simulink model "ESP32_UDP_UART_Bridge"  (R2024b)
settings: Solver=ode4  StartTime=0.0  StopTime=Inf  FixedStep=0.005  RelTol=1e-3  EnableMultiTasking=on
values from neighbouring files (symbols this model uses):
  UDP_DIAG_SOURCE_ID = uint8(1)    [ESP32_UDP_UART_Setup.m]
libraries: arduinowifilib x1, arduinolib x1
(part 2 of 3)

== matlab function ESP32_UDP_UART_Bridge/MATLAB Function3 ==
  data: now_ms input; safe_status_u8 output; fused_status_u8 input; fused_time_u32 input; fused_pose_f32 input; safe_time_u32 output; safe_cmd_u8 output; safe_pose_f32 output
% =========================================================
% ESP32_Link_Safety
% =========================================================
% Zadanie:
%   Realizuje warstwę bezpieczeństwa łącza Vision po fuzji pomiarów.
%   Blok decyduje, czy można dalej jechać, czy należy utrzymać ostatni
%   stan, zmniejszać speed, albo wykonać hard stop.
%
% Wejścia:
%   now_ms          : lokalny czas ESP32 w ms, uint32
%   fused_status_u8 : status z Vision_Measurement_Fusion, 8x1
%   fused_time_u32  : czasy z Vision_Measurement_Fusion, 3x1
%   fused_pose_f32  : pozycja fused, 6x1
%
% Wyjścia:
%   safe_status_u8, 8x1:
%     1 = pose_valid
%     2 = deadman_out
%     3 = move_en_out
%     4 = safe_to_drive
%     5 = hold_mode
%     6 = soft_decay
%     7 = hard_stop
%     8 = source_id
%
%   safe_time_u32, 3x1:
%     1 = seq
%     2 = unity_t_ms
%     3 = link_age_ms
%
%   safe_cmd_u8, 2x1:
%     1 = speed_pct
%     2 = fps_hz
%
%   safe_pose_f32, 6x1:
%     1 = x_m
%     2 = y_m
%     3 = z_m
%     4 = yaw_deg
%     5 = yaw_deg_unwrapped
%     6 = yaw_rate_dps
%
% Metodyka:
%   Jeśli fused_available=1, blok zapamiętuje ostatni poprawny stan.
%   Jeśli przez krótki czas nie ma nowego fused state, blok korzysta
%   z ostatniego zapamiętanego stanu i przechodzi przez tryby:
%      0..75 ms    : normal
%      75..150 ms  : hold last
%      150..250 ms : soft decay, liniowe zmniejszanie speed_pct
%      >250 ms     : hard stop
%
%   Jeśli operator_stop_request=1, hard stop wykonywany jest natychmiast,
%   bez czekania na timeout.
%
% Uwagi:
%   Ten blok nie dekoduje UDP i nie wybiera źródła. Jego zadaniem jest
%   wyłącznie bezpieczne zachowanie wyjścia przy utracie lub zatrzymaniu
%   danych Vision.
% =========================================================

function [safe_status_u8, safe_time_u32, safe_cmd_u8, safe_pose_f32] = ESP32_Link_Safety(now_ms, fused_status_u8, fused_time_u32, fused_pose_f32)
%#codegen

HOLD_NORMAL_MS = uint32(75);
HOLD_LAST_MS   = uint32(150);
SOFT_STOP_MS   = uint32(250);

safe_status_u8 = zeros(8, 1, 'uint8');
safe_time_u32  = zeros(3, 1, 'uint32');
safe_cmd_u8    = zeros(2, 1, 'uint8');
safe_pose_f32  = zeros(6, 1, 'single');

persistent has_last last_ms
persistent last_status last_time last_cmd last_pose

if isempty(has_last)
    has_last = uint8(0);
    last_ms = uint32(0);

    last_status = zeros(8, 1, 'uint8');
    last_time   = zeros(3, 1, 'uint32');
    last_cmd    = zeros(2, 1, 'uint8');
    last_pose   = zeros(6, 1, 'single');
end

fused_available = fused_status_u8(1);
operator_stop_request = fused_status_u8(2);

% Świeży stop operatora: deadman/move_en puszczony
if operator_stop_request ~= 0
    safe_status_u8(7) = uint8(1); % hard_stop
    return;
end

% Aktualizacja ostatniego poprawnego fused state
if fused_available ~= 0
    has_last = uint8(1);
    last_ms = now_ms;

    last_status(:) = fused_status_u8(:);
    last_time(:) = fused_time_u32(:);

    last_cmd(1) = fused_status_u8(4); % speed_pct
    last_cmd(2) = fused_status_u8(5); % fps_hz

    last_pose(:) = fused_pose_f32(:);
end

if has_last == 0
    safe_status_u8(7) = uint8(1); % hard_stop
    return;
end

if now_ms >= last_ms
    link_age_ms = now_ms - last_ms;
else
    link_age_ms = uint32(0);
end

safe_status_u8(1) = uint8(1); % pose_valid
safe_status_u8(2) = uint8(1); % deadman_out
safe_status_u8(3) = uint8(1); % move_en_out
safe_status_u8(8) = last_status(3); % source_id

safe_time_u32(1) = last_time(1); % seq
safe_time_u32(2) = last_time(2); % unity_t_ms
safe_time_u32(3) = link_age_ms;

safe_cmd_u8(1) = last_cmd(1); % speed
safe_cmd_u8(2) = last_cmd(2); % fps

safe_pose_f32(:) = last_pose(:);

if link_age_ms <= HOLD_NORMAL_MS
    safe_status_u8(4) = uint8(1); % safe_to_drive

elseif link_age_ms <= HOLD_LAST_MS
    safe_status_u8(4) = uint8(1);
    safe_status_u8(5) = uint8(1); % hold_mode

elseif link_age_ms <= SOFT_STOP_MS
    safe_status_u8(4) = uint8(1);
    safe_status_u8(6) = uint8(1); % soft_decay

    decay_range = double(SOFT_STOP_MS - HOLD_LAST_MS);
    decay_age = double(link_age_ms - HOLD_LAST_MS);
    factor = 1.0 - decay_age / decay_range;

    if factor < 0.0
        factor = 0.0;
    end

    safe_cmd_u8(1) = uint8(double(last_cmd(1)) * factor);

else
    safe_status_u8(:) = uint8(0);
    safe_status_u8(7) = uint8(1); % hard_stop

    safe_time_u32(1) = last_time(1);
    safe_time_u32(2) = last_time(2);
    safe_time_u32(3) = link_age_ms;

    safe_cmd_u8(:) = uint8(0);
    safe_pose_f32(:) = last_pose(:);
end

== matlab function ESP32_UDP_UART_Bridge/ATU1_UART_Frame_Builder ==
  data: safe_status_u8 input; uart_bytes output; safe_time_u32 input; safe_cmd_u8 input; safe_pose_f32 input; uart_debug_u8 output; uart_crc_u16 output
function [uart_bytes, uart_debug_u8, uart_crc_u16] = ATU1_UART_Frame_Builder(safe_status_u8, safe_time_u32, safe_cmd_u8, safe_pose_f32)
%#codegen
% =========================================================
% ATU1_UART_Frame_Builder
% =========================================================
% Zadanie:
%   Buduje binarną ramkę UART ATU1 wysyłaną z ESP32 do STM32.
%   Ramka zawiera przefiltrowany/fused stan Vision oraz flagi safety.
%
% Format wyjściowy ATU1:
%   bajty 1-2   : header 0xA5 0x5A
%   bajt 3      : version = 1
%   bajt 4      : source_id
%   bajty 5-8   : seq uint32 little-endian
%   bajty 9-12  : unity_t_ms uint32 little-endian
%   bajt 13     : flags
%                 bit0 = pose_valid
%                 bit1 = deadman
%                 bit2 = move_en
%                 bit3 = selected/fused data ok
%                 bit4 = safe_to_drive
%                 bit5 = hold_mode
%                 bit6 = soft_decay
%                 bit7 = hard_stop
%   bajt 14     : speed_pct
%   bajt 15     : fps_hz
%   bajt 16     : reserved
%   bajty 17-20 : x_m single little-endian
%   bajty 21-24 : y_m single little-endian
%   bajty 25-28 : z_m single little-endian
%   bajty 29-32 : yaw_deg_unwrapped single little-endian
%   bajty 33-36 : yaw_rate_dps single little-endian
%   bajty 37-38 : crc16 uint16 little-endian
%
% Wejścia:
%   safe_status_u8, 8x1:
%     1 = pose_valid
%     2 = deadman
%     3 = move_en
%     4 = safe_to_drive
%     5 = hold_mode
%     6 = soft_decay
%     7 = hard_stop
%     8 = source_id
%
%   safe_time_u32, 3x1:
%     1 = seq
%     2 = unity_t_ms
%     3 = link_age_ms, nie jest wysyłane w ATU1 V1
%
%   safe_cmd_u8, 2x1:
%     1 = speed_pct
%     2 = fps_hz
%
%   safe_pose_f32, 6x1:
%     1 = x_m
%     2 = y_m
%     3 = z_m
%     4 = yaw_deg, nie jest wysyłane w ATU1 V1
%     5 = yaw_deg_unwrapped
%     6 = yaw_rate_dps
%
% Wyjścia:
%   uart_bytes, 38x1 uint8:
%     gotowa ramka do wysłania przez UART do STM32
%
%   uart_debug_u8, 8x1 uint8:
%     1 = header byte 1
%     2 = header byte 2
%     3 = version
%     4 = source_id
%     5 = flags
%     6 = speed_pct
%     7 = fps_hz
%     8 = frame length
%
%   uart_crc_u16, 1x1 uint16:
%     CRC16 policzone dla ramki ATU1 po bajtach 1..36
%
% Metodyka:
%   Blok mapuje status safety na pole flags, wpisuje wartości liczbowe
%   w kolejności little-endian, a następnie liczy CRC16 CCITT-FALSE
%   po bajtach 1..36. CRC jest zapisywane w bajtach 37..38.
% =========================================================

uart_bytes    = zeros(38, 1, 'uint8');
uart_debug_u8 = zeros(8, 1, 'uint8');
uart_crc_u16  = zeros(1, 1, 'uint16');

pose_valid    = safe_status_u8(1);
deadman       = safe_status_u8(2);
move_en       = safe_status_u8(3);
safe_to_drive = safe_status_u8(4);
hold_mode     = safe_status_u8(5);
soft_decay    = safe_status_u8(6);
hard_stop     = safe_status_u8(7);
source_id     = safe_status_u8(8);

seq        = safe_time_u32(1);
unity_t_ms = safe_time_u32(2);

speed_pct = safe_cmd_u8(1);
fps_hz    = safe_cmd_u8(2);

x_m = safe_pose_f32(1);
y_m = safe_pose_f32(2);
z_m = safe_pose_f32(3);

yaw_deg_unwrapped = safe_pose_f32(5);
yaw_rate_dps      = safe_pose_f32(6);

% Header
uart_bytes(1) = uint8(165); % 0xA5
uart_bytes(2) = uint8(90);  % 0x5A
uart_bytes(3) = uint8(1);   % version
uart_bytes(4) = source_id;

% seq uint32 little-endian
uart_bytes(5) = uint8(bitand(seq, uint32(255)));
uart_bytes(6) = uint8(bitand(bitshift(seq, -8), uint32(255)));
uart_bytes(7) = uint8(bitand(bitshift(seq, -16), uint32(255)));
uart_bytes(8) = uint8(bitand(bitshift(seq, -24), uint32(255)));

% unity_t_ms uint32 little-endian
uart_bytes(9)  = uint8(bitand(unity_t_ms, uint32(255)));
uart_bytes(10) = uint8(bitand(bitshift(unity_t_ms, -8), uint32(255)));
uart_bytes(11) = uint8(bitand(bitshift(unity_t_ms, -16), uint32(255)));
uart_bytes(12) = uint8(bitand(bitshift(unity_t_ms, -24), uint32(255)));

% Flags
flags = uint8(0);

if pose_valid ~= 0
    flags = bitor(flags, uint8(1));    % bit0 pose_valid
end

if deadman ~= 0
    flags = bitor(flags, uint8(2));    % bit1 deadman
end

if move_en ~= 0
    flags = bitor(flags, uint8(4));    % bit2 move_en
end

if pose_valid ~= 0
    flags = bitor(flags, uint8(8));    % bit3 selected/fused data ok
end

if safe_to_drive ~= 0
    flags = bitor(flags, uint8(16));   % bit4 safe_to_drive
end

if hold_mode ~= 0
    flags = bitor(flags, uint8(32));   % bit5 hold_mode
end

if soft_decay ~= 0
    flags = bitor(flags, uint8(64));   % bit6 soft_decay
end

if hard_stop ~= 0
    flags = bitor(flags, uint8(128));  % bit7 hard_stop
end

uart_bytes(13) = flags;
uart_bytes(14) = speed_pct;
uart_bytes(15) = fps_hz;
uart_bytes(16) = uint8(0); % reserved

% x_m single little-endian
b = typecast(single(x_m), 'uint8');
uart_bytes(17) = b(1);
uart_bytes(18) = b(2);
uart_bytes(19) = b(3);
uart_bytes(20) = b(4);

% y_m single little-endian
b = typecast(single(y_m), 'uint8');
uart_bytes(21) = b(1);
uart_bytes(22) = b(2);
uart_bytes(23) = b(3);
uart_bytes(24) = b(4);

% z_m single little-endian
b = typecast(single(z_m), 'uint8');
uart_bytes(25) = b(1);
uart_bytes(26) = b(2);
uart_bytes(27) = b(3);
uart_bytes(28) = b(4);

% yaw_deg_unwrapped single little-endian
b = typecast(single(yaw_deg_unwrapped), 'uint8');
uart_bytes(29) = b(1);
uart_bytes(30) = b(2);
uart_bytes(31) = b(3);
uart_bytes(32) = b(4);

% yaw_rate_dps single little-endian
b = typecast(single(yaw_rate_dps), 'uint8');
uart_bytes(33) = b(1);
uart_bytes(34) = b(2);
uart_bytes(35) = b(3);
uart_bytes(36) = b(4);

% CRC16 CCITT-FALSE po bajtach 1..36
crc = crc16_ccitt_false_36bytes(uart_bytes);

uart_bytes(37) = uint8(bitand(crc, uint16(255)));
uart_bytes(38) = uint8(bitand(bitshift(crc, -8), uint16(255)));

uart_crc_u16(1) = crc;

% Debug
uart_debug_u8(1) = uart_bytes(1);   % 0xA5
uart_debug_u8(2) = uart_bytes(2);   % 0x5A
uart_debug_u8(3) = uart_bytes(3);   % version
uart_debug_u8(4) = uart_bytes(4);   % source_id
uart_debug_u8(5) = uart_bytes(13);  % flags
uart_debug_u8(6) = uart_bytes(14);  % speed_pct
uart_debug_u8(7) = uart_bytes(15);  % fps_hz
uart_debug_u8(8) = uint8(38);       % frame length
end

function crc = crc16_ccitt_false_36bytes(data)
%#codegen

crc = uint16(65535); % 0xFFFF

for i = 1:36
    crc = bitxor(crc, bitshift(uint16(data(i)), 8));

    for b = 1:8
        if bitand(crc, uint16(32768)) ~= 0 % 0x8000
            crc = bitxor(bitshift(crc, 1), uint16(4129)); % 0x1021
        else
            crc = bitshift(crc, 1);
        end
    end
end
end

== matlab function ESP32_UDP_UART_Bridge/UDP_Link_Diagnostics ==
  data: now_ms input; diag_selected_u32 output; debug_source_id input; portA_udp_data input; portA_udp_size input; portB_udp_data input; portB_udp_size input; diag_selected_u8 output; diag_summary_u32 output; diag_src_u32 output; diag_src_u8 output; diag_port_u32 output
function [diag_selected_u32, diag_selected_u8, diag_summary_u32, diag_src_u32, diag_src_u8, diag_port_u32] = ...
    UDP_Link_Diagnostics(now_ms, debug_source_id, ...
    portA_udp_data, portA_udp_size, ...
    portB_udp_data, portB_udp_size)
%#codegen
% =========================================================
% UDP_Link_Diagnostics
% =========================================================
% Zadanie:
%   Równoległa diagnostyka jakości linku UDP Unity -> ESP32.
%   Blok NIE wpływa na tor sterowania/safety. Czyta surowe dane UDP
%   z PortA/PortB, sam sprawdza ramkę ATB1 i liczy statystyki per source_id.
%
% Wejścia:
%   now_ms          - lokalny czas ESP32/symulacji [ms], uint32
%   debug_source_id - source_id 1..4 wybrany do łatwego podglądu
%   portA_udp_data  - Data z WiFi UDP Receive PortA
%   portA_udp_size  - Size z WiFi UDP Receive PortA
%   portB_udp_data  - Data z WiFi UDP Receive PortB
%   portB_udp_size  - Size z WiFi UDP Receive PortB
%
% Wyjścia:
%   diag_selected_u32 - 20x1 statystyki wybranego source_id
%   diag_selected_u8  - 8x1 flagi wybranego source_id
%   diag_summary_u32  - 12x1 podsumowanie wszystkich source_id
%   diag_src_u32      - 20x4 pełne statystyki source_id 1..4
%   diag_src_u8       - 8x4 pełne flagi source_id 1..4
%   diag_port_u32     - 8x2 statystyki PortA/PortB
%
% Zasada sesji:
%   Jeśli przerwa od ostatniej poprawnej ramki source_id > 2000 ms,
%   zaczynamy nową sesję i NIE liczymy tej przerwy jako packet loss.
%
% Zasada świeżości:
%   Źródło jest fresh, jeśli age_ms <= 300 ms.
%
% Format ATB1:
%   42 B, header A1 1A, version=1, source_id=1..4,
%   CRC16/CCITT-FALSE po bajtach 1..40.
% =========================================================

FRESH_MS = uint32(300);
SESSION_GAP_MS = uint32(2000);

persistent src_u32 src_u8 port_u32

if isempty(src_u32)
    src_u32  = zeros(20, 4, 'uint32');
    src_u8   = zeros(8, 4, 'uint8');
    port_u32 = zeros(8, 2, 'uint32');
end

[src_u32, src_u8, port_u32] = update_one_port(now_ms, uint8(1), portA_udp_data, portA_udp_size, src_u32, src_u8, port_u32, SESSION_GAP_MS);
[src_u32, src_u8, port_u32] = update_one_port(now_ms, uint8(2), portB_udp_data, portB_udp_size, src_u32, src_u8, port_u32, SESSION_GAP_MS);

% Aktualizacja age/fresh/in_session dla każdego source_id
for i = 1:4
    if src_u8(1, i) ~= uint8(0)
        last_rx_ms = src_u32(9, i);

        if now_ms >= last_rx_ms
            age_ms = now_ms - last_rx_ms;
        else
            age_ms = uint32(0);
        end

        src_u32(19, i) = age_ms; % age_ms

        if age_ms <= FRESH_MS
            src_u8(2, i) = uint8(1); % fresh_300ms
        else
            src_u8(2, i) = uint8(0);
        end

        if age_ms <= SESSION_GAP_MS
            src_u8(3, i) = uint8(1); % in_session
        else
            src_u8(3, i) = uint8(0);
        end
    end
end

% Summary
diag_summary_u32 = zeros(12, 1, 'uint32');

total_rx_ok = uint32(0);
total_lost = uint32(0);
total_crc_bad = uint32(0);
total_dup = uint32(0);
sources_seen_mask = uint32(0);
fresh_sources_mask = uint32(0);
max_gap_all = uint32(0);
worst_age = uint32(0);
fresh_count = uint32(0);
total_sessions = uint32(0);

for i = 1:4
    total_rx_ok = total_rx_ok + src_u32(1, i);
    total_crc_bad = total_crc_bad + src_u32(2, i);
    total_lost = total_lost + src_u32(3, i);
    total_dup = total_dup + src_u32(4, i);
    total_sessions = total_sessions + src_u32(15, i);

    if src_u8(1, i) ~= uint8(0)
        sources_seen_mask = bitor(sources_seen_mask, bitshift(uint32(1), i - 1));
    end

    if src_u8(2, i) ~= uint8(0)
        fresh_sources_mask = bitor(fresh_sources_mask, bitshift(uint32(1), i - 1));
        fresh_count = fresh_count + uint32(1);
    end

    if src_u32(11, i) > max_gap_all
        max_gap_all = src_u32(11, i);
    end

    if src_u32(19, i) > worst_age
        worst_age = src_u32(19, i);
    end
end

diag_summary_u32(1) = total_rx_ok;
diag_summary_u32(2) = total_lost;
diag_summary_u32(3) = total_crc_bad;
diag_summary_u32(4) = total_dup;
diag_summary_u32(5) = sources_seen_mask;
diag_summary_u32(6) = fresh_sources_mask;
diag_summary_u32(7) = max_gap_all;
diag_summary_u32(8) = worst_age;

den = total_rx_ok + total_lost;
if den > uint32(0)
    diag_summary_u32(9) = uint32((double(total_lost) * 1000.0) / double(den)); % total_loss_permille
else
    diag_summary_u32(9) = uint32(0);
end

diag_summary_u32(10) = fresh_count;
diag_summary_u32(11) = total_sessions;
diag_summary_u32(12) = uint32(0);

% Wybór source_id do prostego podglądu
sid = debug_source_id;

if sid < uint8(1) || sid > uint8(4)
    sid = uint8(1);
end

idx = double(sid);

diag_selected_u32 = src_u32(:, idx);
diag_selected_u8  = src_u8(:, idx);

diag_src_u32 = src_u32;
diag_src_u8  = src_u8;
diag_port_u32 = port_u32;
end

function [src_u32, src_u8, port_u32] = update_one_port(now_ms, port_id, udp_data, udp_size, src_u32, src_u8, port_u32, SESSION_GAP_MS)
%#codegen

ATB1_LEN = uint32(42);

p = double(port_id);
payload_len = uint32(udp_size);

% Brak datagramu w tym kroku - nie liczymy tego jako błąd.
if payload_len == uint32(0)
    return;
end

% Ignoruj własne ramki diagnostyczne ATD1, jeśli broadcast wróci do odbiornika.
% ATD1: len=96, header AD D1.
if payload_len >= uint32(2)
    if udp_data(1) == uint8(173) && udp_data(2) == uint8(209)
        return;
    end
end

% Port stats:
% 1 = frame_seen
% 2 = len_bad
% 3 = header_bad
% 4 = version_bad
% 5 = source_bad
% 6 = crc_bad_known_or_unknown
% 7 = ok_known
% 8 = reserved
port_u32(1, p) = port_u32(1, p) + uint32(1);

% Length check
if payload_len ~= ATB1_LEN
    port_u32(2, p) = port_u32(2, p) + uint32(1);
    return;
end

% Header A1 1A
if udp_data(1) ~= uint8(161) || udp_data(2) ~= uint8(26)
    port_u32(3, p) = port_u32(3, p) + uint32(1);
    return;
end

% Version
if udp_data(3) ~= uint8(1)
    port_u32(4, p) = port_u32(4, p) + uint32(1);
    return;
end

source_id = udp_data(4);

if source_id < uint8(1) || source_id > uint8(4)
    port_u32(5, p) = port_u32(5, p) + uint32(1);
    return;
end

idx = double(source_id);

seq        = read_u32_le(udp_data, 5);
unity_t_ms = read_u32_le(udp_data, 9);

flags = udp_data(13);

valid   = uint8(bitand(flags, uint8(1)) ~= 0);
deadman = uint8(bitand(flags, uint8(2)) ~= 0);
move_en = uint8(bitand(flags, uint8(4)) ~= 0);

crc_rx   = read_u16_le(udp_data, 41);
crc_calc = crc16_ccitt_false_n(udp_data, uint32(40));

if crc_rx ~= crc_calc
    src_u32(2, idx) = src_u32(2, idx) + uint32(1); % crc_bad_total
    src_u8(8, idx) = uint8(6);                     % last_error_code = crc_bad
    port_u32(6, p) = port_u32(6, p) + uint32(1);
    return;
end

% Od tego miejsca ramka ma poprawny header/version/source/CRC.
port_u32(7, p) = port_u32(7, p) + uint32(1); % ok_known

seen_before = src_u8(1, idx) ~= uint8(0);

gap_ms = uint32(0);
new_session = false;

if seen_before
    last_rx_ms = src_u32(9, idx);

    if now_ms >= last_rx_ms
        gap_ms = now_ms - last_rx_ms;
    else
        gap_ms = uint32(0);
    end

    if gap_ms > SESSION_GAP_MS
        new_session = true;
    end
else
    new_session = true;
end

% Start nowej sesji.
% Długa przerwa >2000 ms nie jest liczona jako packet loss.
if new_session
    src_u32(15, idx) = src_u32(15, idx) + uint32(1); % session_id
    src_u32(16, idx) = uint32(0); % session_rx_ok
    src_u32(17, idx) = uint32(0); % session_lost
    src_u32(18, idx) = uint32(0); % session_max_gap_ms
    gap_ms = uint32(0);
else
    last_seq = src_u32(8, idx);

    if seq > last_seq + uint32(1)
        lost = seq - last_seq - uint32(1);
        src_u32(3, idx)  = src_u32(3, idx) + lost; % seq_lost_total
        src_u32(17, idx) = src_u32(17, idx) + lost; % session_lost
    elseif seq <= last_seq
        % Duplikat albo stara ramka.
        src_u32(1, idx) = src_u32(1, idx) + uint32(1); % rx_ok_total, bo ramka CRC OK
        src_u32(4, idx) = src_u32(4, idx) + uint32(1); % duplicate_or_old
        src_u32(9, idx) = now_ms;
        src_u32(10, idx) = gap_ms;

        if gap_ms > src_u32(11, idx)
            src_u32(11, idx) = gap_ms;
        end

        if gap_ms > src_u32(18, idx)
            src_u32(18, idx) = gap_ms;
        end

        if src_u32(12, idx) == uint32(0)
            src_u32(12, idx) = gap_ms;
        else
            src_u32(12, idx) = uint32((double(src_u32(12, idx))*7.0 + double(gap_ms)) / 8.0);
        end

        src_u8(1, idx) = uint8(1); % source_seen
        src_u8(7, idx) = port_id;
        src_u8(8, idx) = uint8(7); % duplicate_or_old
        return;
    end

    src_u32(10, idx) = gap_ms; % last_gap_ms

    if gap_ms > src_u32(11, idx)
        src_u32(11, idx) = gap_ms; % max_gap_ms
    end

    if gap_ms > src_u32(18, idx)
        src_u32(18, idx) = gap_ms; % session_max_gap_ms
    end

    if src_u32(12, idx) == uint32(0)
        src_u32(12, idx) = gap_ms;
    else
        src_u32(12, idx) = uint32((double(src_u32(12, idx))*7.0 + double(gap_ms)) / 8.0);
    end
end

% Poprawna, nowa ramka.
src_u32(1, idx)  = src_u32(1, idx) + uint32(1); % rx_ok_total
src_u32(16, idx) = src_u32(16, idx) + uint32(1); % session_rx_ok

if valid ~= uint8(0)
    src_u32(5, idx) = src_u32(5, idx) + uint32(1);
end

if deadman ~= uint8(0)
    src_u32(6, idx) = src_u32(6, idx) + uint32(1);
end

if move_en ~= uint8(0)
    src_u32(7, idx) = src_u32(7, idx) + uint32(1);
end

src_u32(8, idx) = seq;          % last_seq
src_u32(9, idx) = now_ms;       % last_rx_ms
src_u32(20, idx) = unity_t_ms;  % last_unity_t_ms

den_loss = src_u32(1, idx) + src_u32(3, idx);
if den_loss > uint32(0)
    src_u32(13, idx) = uint32((double(src_u32(3, idx)) * 1000.0) / double(den_loss));
else
    src_u32(13, idx) = uint32(0);
end

if src_u32(1, idx) > uint32(0)
    src_u32(14, idx) = uint32((double(src_u32(5, idx)) * 100.0) / double(src_u32(1, idx)));
else
    src_u32(14, idx) = uint32(0);
end

src_u8(1, idx) = uint8(1); % source_seen
src_u8(4, idx) = valid;
src_u8(5, idx) = deadman;
src_u8(6, idx) = move_en;
src_u8(7, idx) = port_id;
src_u8(8, idx) = uint8(1); % OK
end

function y = read_u16_le(data, idx)
%#codegen
b0 = uint16(data(idx));
b1 = uint16(data(idx + 1));
y = bitor(b0, bitshift(b1, 8));
end

function y = read_u32_le(data, idx)
%#codegen
b0 = uint32(data(idx));
b1 = uint32(data(idx + 1));
b2 = uint32(data(idx + 2));
b3 = uint32(data(idx + 3));

y = bitor(b0, bitshift(b1, 8));
y = bitor(y, bitshift(b2, 16));
y = bitor(y, bitshift(b3, 24));
end

function crc = crc16_ccitt_false_n(data, n)
%#codegen

crc = uint16(65535); % 0xFFFF

for i = 1:n
    crc = bitxor(crc, bitshift(uint16(data(i)), 8));

    for b = 1:8
        if bitand(crc, uint16(32768)) ~= 0 % 0x8000
            crc = bitxor(bitshift(crc, 1), uint16(4129)); % 0x1021
        else
            crc = bitshift(crc, 1);
        end
    end
end
end

== matlab function ESP32_UDP_UART_Bridge/MATLAB Function4 ==
  data: now_ms input; uart_bytes input; diag_tx_bytes output; diag_src_u32 input; diag_src_u8 input; diag_tx_send output
function [diag_tx_bytes, diag_tx_send] = ...
    UDP_Diag_TX_Builder( ...
        now_ms,...
        uart_bytes,  ...
        diag_src_u32, ...
        diag_src_u8)
%#codegen
% =========================================================
% UDP_Diag_TX_Builder
% =========================================================
% Co 5 sekund wysyła dwie osobne ramki:
%   source_id = 1
%   source_id = 2
%
% Pierwsze 96 bajtów:
%   standardowa diagnostyka ATD1
%
% Bajty od 97 do końca:
%   dokładna kopia wektora uart_bytes wysyłanego do STM32
%
% Całkowita długość datagramu:
%   96 + numel(uart_bytes)
%
% Uwaga:
% Jest to snapshot bieżącej ramki UART wykonywany raz na
% 5 sekund, a nie kopia każdej transmisji UART.
% =========================================================

TX_PERIOD_MS = uint32(5000);

ATD1_LENGTH = 96;
UART_LENGTH = numel(uart_bytes);
TOTAL_LENGTH = ATD1_LENGTH + UART_LENGTH;

diag_tx_bytes = zeros(TOTAL_LENGTH, 1, 'uint8');
diag_tx_send = uint8(0);

persistent last_cycle_ms
persistent tx_counter
persistent pending_source2
persistent initialized

if isempty(initialized)
    last_cycle_ms = now_ms;
    tx_counter = uint32(0);
    pending_source2 = uint8(0);
    initialized = uint8(1);
end

% Obsługa resetu lub zawinięcia czasu
if now_ms < last_cycle_ms
    last_cycle_ms = now_ms;
    pending_source2 = uint8(0);
end

% Source 2 wysyłamy w kolejnym kroku modelu po source 1
if pending_source2 ~= uint8(0)

    source_id = uint8(2);
    pending_source2 = uint8(0);

% Rozpoczęcie nowego cyklu diagnostycznego
elseif (now_ms - last_cycle_ms) >= TX_PERIOD_MS

    last_cycle_ms = now_ms;

    source_id = uint8(1);
    pending_source2 = uint8(1);

else
    return;
end

idx = double(source_id);

tx_counter = tx_counter + uint32(1);
diag_tx_send = uint8(1);

% =========================================================
% ATD1: bajty 1–96
% =========================================================

% Header ATD1
diag_tx_bytes(1) = uint8(173); % 0xAD
diag_tx_bytes(2) = uint8(209); % 0xD1
diag_tx_bytes(3) = uint8(1);   % version
diag_tx_bytes(4) = source_id;

% Czas ESP32 i licznik ramek diagnostycznych
diag_tx_bytes = write_u32_le( ...
    diag_tx_bytes, 5, now_ms);

diag_tx_bytes = write_u32_le( ...
    diag_tx_bytes, 9, tx_counter);

% Statystyki source_id
diag_tx_bytes = write_u32_le( ...
    diag_tx_bytes, 13, diag_src_u32(1, idx));

diag_tx_bytes = write_u32_le( ...
    diag_tx_bytes, 17, diag_src_u32(2, idx));

diag_tx_bytes = write_u32_le( ...
    diag_tx_bytes, 21, diag_src_u32(3, idx));

diag_tx_bytes = write_u32_le( ...
    diag_tx_bytes, 25, diag_src_u32(4, idx));

diag_tx_bytes = write_u32_le( ...
    diag_tx_bytes, 29, diag_src_u32(5, idx));

diag_tx_bytes = write_u32_le( ...
    diag_tx_bytes, 33, diag_src_u32(6, idx));

diag_tx_bytes = write_u32_le( ...
    diag_tx_bytes, 37, diag_src_u32(7, idx));

diag_tx_bytes = write_u32_le( ...
    diag_tx_bytes, 41, diag_src_u32(8, idx));

diag_tx_bytes = write_u32_le( ...
    diag_tx_bytes, 45, diag_src_u32(10, idx));

diag_tx_bytes = write_u32_le( ...
    diag_tx_bytes, 49, diag_src_u32(11, idx));

diag_tx_bytes = write_u32_le( ...
    diag_tx_bytes, 53, diag_src_u32(12, idx));

diag_tx_bytes = write_u32_le( ...
    diag_tx_bytes, 57, diag_src_u32(13, idx));

diag_tx_bytes = write_u32_le( ...
    diag_tx_bytes, 61, diag_src_u32(14, idx));

diag_tx_bytes = write_u32_le( ...
    diag_tx_bytes, 65, diag_src_u32(15, idx));

diag_tx_bytes = write_u32_le( ...
    diag_tx_bytes, 69, diag_src_u32(16, idx));

diag_tx_bytes = write_u32_le( ...
    diag_tx_bytes, 73, diag_src_u32(17, idx));

diag_tx_bytes = write_u32_le( ...
    diag_tx_bytes, 77, diag_src_u32(18, idx));

diag_tx_bytes = write_u32_le( ...
    diag_tx_bytes, 81, diag_src_u32(19, idx));

diag_tx_bytes = write_u32_le( ...
    diag_tx_bytes, 85, diag_src_u32(20, idx));

% Flagi source_id
diag_tx_bytes(89) = diag_src_u8(1, idx);
diag_tx_bytes(90) = diag_src_u8(2, idx);
diag_tx_bytes(91) = diag_src_u8(3, idx);
diag_tx_bytes(92) = diag_src_u8(4, idx);
diag_tx_bytes(93) = diag_src_u8(5, idx);
diag_tx_bytes(94) = diag_src_u8(6, idx);
diag_tx_bytes(95) = diag_src_u8(7, idx);
diag_tx_bytes(96) = diag_src_u8(8, idx);

% =========================================================
% Kopia UART: bajty od 97 do końca
% =========================================================
%
% Kopiujemy dokładnie cały stałowymiarowy wektor, który
% trafia do bloku Serial Transmit.
%
% Pętla jest bezpieczna dla code generation i jednoznacznie
% utrzymuje stałe rozmiary sygnałów.
% =========================================================

for k = 1:UART_LENGTH
    diag_tx_bytes(ATD1_LENGTH + k) = ...
        uint8(uart_bytes(k));
end

end


function data = write_u32_le(data, idx, val)
%#codegen

value = uint32(val);

data(idx) = ...
    uint8(bitand(value, uint32(255)));

data(idx + 1) = ...
    uint8(bitand( ...
        bitshift(value, -8), ...
        uint32(255)));

data(idx + 2) = ...
    uint8(bitand( ...
        bitshift(value, -16), ...
        uint32(255)));

data(idx + 3) = ...
    uint8(bitand( ...
        bitshift(value, -24), ...
        uint32(255)));

end

== matlab function ESP32_UDP_UART_Bridge/MATLAB Function5 ==
  data: uart_bytes input; valid output; deadman output; move_en output; fused_available output; safe_to_drive output; hard_stop output; flags output; source_id output; seq output
function [valid, deadman, move_en, fused_available, ...
          safe_to_drive, hard_stop, flags, source_id, seq] = ...
          ATU_Output_View(uart_bytes)
%#codegen
% Dekodowanie faktycznej ramki przekazywanej do UART STM32.

valid = uint8(0);
deadman = uint8(0);
move_en = uint8(0);
fused_available = uint8(0);
safe_to_drive = uint8(0);
hard_stop = uint8(0);

flags = uint8(0);
source_id = uint8(0);
seq = uint32(0);

if numel(uart_bytes) < 16
    return;
end

% Binarny nagłówek A5 5A
if uart_bytes(1) ~= uint8(165) || ...
   uart_bytes(2) ~= uint8(90)
    return;
end

source_id = uint8(uart_bytes(4));

seq = ...
    uint32(uart_bytes(5)) + ...
    bitshift(uint32(uart_bytes(6)), 8) + ...
    bitshift(uint32(uart_bytes(7)), 16) + ...
    bitshift(uint32(uart_bytes(8)), 24);

% Bajt 13 ramki UART
flags = uint8(uart_bytes(13));

valid           = uint8(bitget(flags, 1));
deadman         = uint8(bitget(flags, 2));
move_en         = uint8(bitget(flags, 3));
fused_available = uint8(bitget(flags, 4));
safe_to_drive   = uint8(bitget(flags, 5));

% 0x80 — hard stop
hard_stop = uint8(bitget(flags, 8));
end

== matlab function ESP32_UDP_UART_Bridge/Subsystem/Wrap_Yaw_For_Plot ==
  data: u input; y output
function y = Wrap_Yaw_For_Plot(u)
%#codegen
% Zawija kąt w stopniach do zakresu -180...180.
% Używane tylko do wykresów, niekoniecznie do regulatora.

y = single(mod(single(u) + single(180), single(360)) - single(180));

end

== matlab function ESP32_UDP_UART_Bridge/Subsystem/Wrap_Yaw_For_Plot1 ==
  data: u input; y output
function y = Wrap_Yaw_For_Plot(u)
%#codegen
% Zawija kąt w stopniach do zakresu -180...180.
% Używane tylko do wykresów, niekoniecznie do regulatora.

y = single(mod(single(u) + single(180), single(360)) - single(180));

end

== matlab function ESP32_UDP_UART_Bridge/Subsystem/Wrap_Yaw_For_Plot2 ==
  data: u input; y output
function y = Wrap_Yaw_For_Plot(u)
%#codegen
% Zawija kąt w stopniach do zakresu -180...180.
% Używane tylko do wykresów, niekoniecznie do regulatora.

y = single(mod(single(u) + single(180), single(360)) - single(180));

end

== matlab function ESP32_UDP_UART_Bridge/Subsystem/Wrap_Yaw_For_Plot3 ==
  data: u input; y output
function y = Wrap_Yaw_For_Plot(u)
%#codegen
% Zawija kąt w stopniach do zakresu -180...180.
% Używane tylko do wykresów, niekoniecznie do regulatora.

y = single(mod(single(u) + single(180), single(360)) - single(180));

end

== matlab function ESP32_UDP_UART_Bridge/Subsystem/Wrap_Yaw_For_Plot4 ==
  data: u input; y output
function y = Wrap_Yaw_For_Plot(u)
%#codegen
% Zawija kąt w stopniach do zakresu -180...180.
% Używane tylko do wykresów, niekoniecznie do regulatora.

y = single(mod(single(u) + single(180), single(360)) - single(180));

end

== matlab function ESP32_UDP_UART_Bridge/Subsystem/Wrap_Yaw_For_Plot5 ==
  data: u input; y output
function y = Wrap_Yaw_For_Plot(u)
%#codegen
% Zawija kąt w stopniach do zakresu -180...180.
% Używane tylko do wykresów, niekoniecznie do regulatora.

y = single(mod(single(u) + single(180), single(360)) - single(180));

end

== matlab function ESP32_UDP_UART_Bridge/UDP_Binary_Frame_Decode_B ==
  data: udp_data input; rx_status_u8 output; udp_size input; rx_time_u32 output; rx_pose_f32 output; rx_crc_u16 output
% =========================================================
% ATB1_Decode
% =========================================================
% Zadanie:
%   Dekoduje binarną ramkę UDP ATB1 wysyłaną z Unity/Android
%   do ESP32. Blok nie interpretuje, z którego portu UDP przyszła
%   ramka — zajmuje się tylko zawartością datagramu.
%
% Format wejściowy ATB1:
%   bajty 1-2   : header 0xA1 0x1A
%   bajt 3      : version = 1
%   bajt 4      : source_id, zakres 1..4
%   bajty 5-8   : seq uint32 little-endian
%   bajty 9-12  : unity_t_ms uint32 little-endian
%   bajt 13     : flags
%                 bit0 = valid
%                 bit1 = deadman
%                 bit2 = move_en
%   bajt 14     : speed_pct uint8
%   bajt 15     : fps_hz uint8
%   bajt 16     : reserved
%   bajty 17-20 : x_m single little-endian
%   bajty 21-24 : y_m single little-endian
%   bajty 25-28 : z_m single little-endian
%   bajty 29-32 : yaw_deg single little-endian
%   bajty 33-36 : yaw_deg_unwrapped single little-endian
%   bajty 37-40 : yaw_rate_dps single little-endian
%   bajty 41-42 : crc16 uint16 little-endian
%
% Wyjścia:
%   rx_status_u8, 8x1:
%     1 = frame_ok
%     2 = source_id
%     3 = valid
%     4 = deadman
%     5 = move_en
%     6 = speed_pct
%     7 = fps_hz
%     8 = reserved
%
%   rx_time_u32, 2x1:
%     1 = seq
%     2 = unity_t_ms
%
%   rx_pose_f32, 6x1:
%     1 = x_m
%     2 = y_m
%     3 = z_m
%     4 = yaw_deg
%     5 = yaw_deg_unwrapped
%     6 = yaw_rate_dps
%
%   rx_crc_u16, 2x1:
%     1 = crc_rx
%     2 = crc_calc
%
% Metodyka:
%   Blok najpierw sprawdza minimalną długość, header, wersję oraz
%   source_id. Następnie odczytuje pola little-endian, liczy CRC16
%   CCITT-FALSE po bajtach 1..40 i ustawia frame_ok=1 tylko wtedy,
%   gdy CRC odebrane zgadza się z CRC policzonym lokalnie.
%
% Uwagi:
%   Jeśli frame_ok=0, dalsza logika ignoruje pakiet.
%   rx_crc_u16 jest wyjściem diagnostycznym; samo CRC jest już użyte
%   wewnątrz tego bloku do wyznaczenia frame_ok.
% =========================================================

function [rx_status_u8, rx_time_u32, rx_pose_f32, rx_crc_u16] = ATB1_Decode(udp_data, udp_size)
%#codegen

rx_status_u8 = zeros(8, 1, 'uint8');
rx_time_u32  = zeros(2, 1, 'uint32');
rx_pose_f32  = zeros(6, 1, 'single');
rx_crc_u16   = zeros(2, 1, 'uint16');

% ATB1 Unity -> ESP32
% 42 bytes, header A1 1A, little-endian

if udp_size < 42
    return;
end

% Header A1 1A
if udp_data(1) ~= uint8(161)   % 0xA1
    return;
end

if udp_data(2) ~= uint8(26)    % 0x1A
    return;
end

% Version = 1
if udp_data(3) ~= uint8(1)
    return;
end

source_id = udp_data(4);

if source_id < uint8(1) || source_id > uint8(4)
    return;
end

seq        = read_u32_le(udp_data, 5);
unity_t_ms = read_u32_le(udp_data, 9);

flags = udp_data(13);

valid   = uint8(bitand(flags, uint8(1)) ~= 0);
deadman = uint8(bitand(flags, uint8(2)) ~= 0);
move_en = uint8(bitand(flags, uint8(4)) ~= 0);

speed_pct = udp_data(14);
fps_hz    = udp_data(15);

x_m = read_f32_le(udp_data, 17);
y_m = read_f32_le(udp_data, 21);
z_m = read_f32_le(udp_data, 25);

yaw_deg           = read_f32_le(udp_data, 29);
yaw_deg_unwrapped = read_f32_le(udp_data, 33);
yaw_rate_dps      = read_f32_le(udp_data, 37);

crc_rx   = read_u16_le(udp_data, 41);
crc_calc = crc16_ccitt_false_40bytes(udp_data);

rx_crc_u16(1) = crc_rx;
rx_crc_u16(2) = crc_calc;

frame_ok = uint8(0);

if crc_rx == crc_calc
    frame_ok = uint8(1);
end

rx_status_u8(1) = frame_ok;
rx_status_u8(2) = source_id;
rx_status_u8(3) = valid;
rx_status_u8(4) = deadman;
rx_status_u8(5) = move_en;
rx_status_u8(6) = speed_pct;
rx_status_u8(7) = fps_hz;
rx_status_u8(8) = uint8(0); % reserved, nie port

rx_time_u32(1) = seq;
rx_time_u32(2) = unity_t_ms;

rx_pose_f32(1) = x_m;
rx_pose_f32(2) = y_m;
rx_pose_f32(3) = z_m;
rx_pose_f32(4) = yaw_deg;
rx_pose_f32(5) = yaw_deg_unwrapped;
rx_pose_f32(6) = yaw_rate_dps;
end

function y = read_u16_le(data, idx)
%#codegen
b0 = uint16(data(idx));
b1 = uint16(data(idx + 1));
y = bitor(b0, bitshift(b1, 8));
end

function y = read_u32_le(data, idx)
%#codegen
b0 = uint32(data(idx));
b1 = uint32(data(idx + 1));
b2 = uint32(data(idx + 2));
b3 = uint32(data(idx + 3));

y = bitor(b0, bitshift(b1, 8));
y = bitor(y, bitshift(b2, 16));
y = bitor(y, bitshift(b3, 24));
end

function y = read_f32_le(data, idx)
%#codegen
bytes = zeros(1, 4, 'uint8');

bytes(1) = data(idx);
bytes(2) = data(idx + 1);
bytes(3) = data(idx + 2);
bytes(4) = data(idx + 3);

y = typecast(bytes, 'single');
end

function crc = crc16_ccitt_false_40bytes(data)
%#codegen

crc = uint16(65535); % 0xFFFF

for i = 1:40
    crc = bitxor(crc, bitshift(uint16(data(i)), 8));

    for b = 1:8
        if bitand(crc, uint16(32768)) ~= 0 % 0x8000
            crc = bitxor(bitshift(crc, 1), uint16(4129)); % 0x1021
        else
            crc = bitshift(crc, 1);
        end
    end
end
end

== matlab function ESP32_UDP_UART_Bridge/UDP_Binary_Frame_Decode_A ==
  data: udp_data input; rx_status_u8 output; udp_size input; rx_time_u32 output; rx_pose_f32 output; rx_crc_u16 output
% =========================================================
% ATB1_Decode
% =========================================================
% Zadanie:
%   Dekoduje binarną ramkę UDP ATB1 wysyłaną z Unity/Android
%   do ESP32. Blok nie interpretuje, z którego portu UDP przyszła
%   ramka — zajmuje się tylko zawartością datagramu.
%
% Format wejściowy ATB1:
%   bajty 1-2   : header 0xA1 0x1A
%   bajt 3      : version = 1
%   bajt 4      : source_id, zakres 1..4
%   bajty 5-8   : seq uint32 little-endian
%   bajty 9-12  : unity_t_ms uint32 little-endian
%   bajt 13     : flags
%                 bit0 = valid
%                 bit1 = deadman
%                 bit2 = move_en
%   bajt 14     : speed_pct uint8
%   bajt 15     : fps_hz uint8
%   bajt 16     : reserved
%   bajty 17-20 : x_m single little-endian
%   bajty 21-24 : y_m single little-endian
%   bajty 25-28 : z_m single little-endian
%   bajty 29-32 : yaw_deg single little-endian
%   bajty 33-36 : yaw_deg_unwrapped single little-endian
%   bajty 37-40 : yaw_rate_dps single little-endian
%   bajty 41-42 : crc16 uint16 little-endian
%
% Wyjścia:
%   rx_status_u8, 8x1:
%     1 = frame_ok
%     2 = source_id
%     3 = valid
%     4 = deadman
%     5 = move_en
%     6 = speed_pct
%     7 = fps_hz
%     8 = reserved
%
%   rx_time_u32, 2x1:
%     1 = seq
%     2 = unity_t_ms
%
%   rx_pose_f32, 6x1:
%     1 = x_m
%     2 = y_m
%     3 = z_m
%     4 = yaw_deg
%     5 = yaw_deg_unwrapped
%     6 = yaw_rate_dps
%
%   rx_crc_u16, 2x1:
%     1 = crc_rx
%     2 = crc_calc
%
% Metodyka:
%   Blok najpierw sprawdza minimalną długość, header, wersję oraz
%   source_id. Następnie odczytuje pola little-endian, liczy CRC16
%   CCITT-FALSE po bajtach 1..40 i ustawia frame_ok=1 tylko wtedy,
%   gdy CRC odebrane zgadza się z CRC policzonym lokalnie.
%
% Uwagi:
%   Jeśli frame_ok=0, dalsza logika ignoruje pakiet.
%   rx_crc_u16 jest wyjściem diagnostycznym; samo CRC jest już użyte
%   wewnątrz tego bloku do wyznaczenia frame_ok.
% =========================================================


function [rx_status_u8, rx_time_u32, rx_pose_f32, rx_crc_u16] = ATB1_Decode(udp_data, udp_size)
%#codegen

rx_status_u8 = zeros(8, 1, 'uint8');
rx_time_u32  = zeros(2, 1, 'uint32');
rx_pose_f32  = zeros(6, 1, 'single');
rx_crc_u16   = zeros(2, 1, 'uint16');

% ATB1 Unity -> ESP32
% 42 bytes, header A1 1A, little-endian

if udp_size < 42
    return;
end

% Header A1 1A
if udp_data(1) ~= uint8(161)   % 0xA1
    return;
end

if udp_data(2) ~= uint8(26)    % 0x1A
    return;
end

% Version = 1
if udp_data(3) ~= uint8(1)
    return;
end

source_id = udp_data(4);

if source_id < uint8(1) || source_id > uint8(4)
    return;
end

seq        = read_u32_le(udp_data, 5);
unity_t_ms = read_u32_le(udp_data, 9);

flags = udp_data(13);

valid   = uint8(bitand(flags, uint8(1)) ~= 0);
deadman = uint8(bitand(flags, uint8(2)) ~= 0);
move_en = uint8(bitand(flags, uint8(4)) ~= 0);

speed_pct = udp_data(14);
fps_hz    = udp_data(15);

x_m = read_f32_le(udp_data, 17);
y_m = read_f32_le(udp_data, 21);
z_m = read_f32_le(udp_data, 25);

yaw_deg           = read_f32_le(udp_data, 29);
yaw_deg_unwrapped = read_f32_le(udp_data, 33);
yaw_rate_dps      = read_f32_le(udp_data, 37);

crc_rx   = read_u16_le(udp_data, 41);
crc_calc = crc16_ccitt_false_40bytes(udp_data);

rx_crc_u16(1) = crc_rx;
rx_crc_u16(2) = crc_calc;

frame_ok = uint8(0);

if crc_rx == crc_calc
    frame_ok = uint8(1);
end

rx_status_u8(1) = frame_ok;
rx_status_u8(2) = source_id;
rx_status_u8(3) = valid;
rx_status_u8(4) = deadman;
rx_status_u8(5) = move_en;
rx_status_u8(6) = speed_pct;
rx_status_u8(7) = fps_hz;
rx_status_u8(8) = uint8(0); % reserved, nie port

rx_time_u32(1) = seq;
rx_time_u32(2) = unity_t_ms;

rx_pose_f32(1) = x_m;
rx_pose_f32(2) = y_m;
rx_pose_f32(3) = z_m;
rx_pose_f32(4) = yaw_deg;
rx_pose_f32(5) = yaw_deg_unwrapped;
rx_pose_f32(6) = yaw_rate_dps;
end

function y = read_u16_le(data, idx)
%#codegen
b0 = uint16(data(idx));
b1 = uint16(data(idx + 1));
y = bitor(b0, bitshift(b1, 8));
end

function y = read_u32_le(data, idx)
%#codegen
b0 = uint32(data(idx));
b1 = uint32(data(idx + 1));
b2 = uint32(data(idx + 2));
b3 = uint32(data(idx + 3));

y = bitor(b0, bitshift(b1, 8));
y = bitor(y, bitshift(b2, 16));
y = bitor(y, bitshift(b3, 24));
end

function y = read_f32_le(data, idx)
%#codegen
bytes = zeros(1, 4, 'uint8');

bytes(1) = data(idx);
bytes(2) = data(idx + 1);
bytes(3) = data(idx + 2);
bytes(4) = data(idx + 3);

y = typecast(bytes, 'single');
end

function crc = crc16_ccitt_false_40bytes(data)
%#codegen

crc = uint16(65535); % 0xFFFF

for i = 1:40
    crc = bitxor(crc, bitshift(uint16(data(i)), 8));

    for b = 1:8
        if bitand(crc, uint16(32768)) ~= 0 % 0x8000
            crc = bitxor(bitshift(crc, 1), uint16(4129)); % 0x1021
        else
            crc = bitshift(crc, 1);
        end
    end
end
end
